simulink model "SCIM08"  (R2016a)
settings: Solver=FixedStepAuto  StartTime=0.0  StopTime=0.2  FixedStep=0.0001  RelTol=1e-3
values from neighbouring files (symbols this model uses):
  Lm = 0.1271    [motor4_workspace.mat]    (also in motor_wrapper.m = obj.Lm; scim_verifier.m = obj.motor.getLm(); setMotorParams.m; stationary_class.m = obj.Lm)
  Lr = 0.2744    [motor4_workspace.mat]    (also in motor_wrapper.m = obj.Lr; scim_verifier.m = obj.motor.getLr(); setMotorParams.m; stationary_class.m = obj.Lr)
  Ls = 0.2744    [motor4_workspace.mat]    (also in motor_wrapper.m = obj.Ls; scim_verifier.m = obj.motor.getLs(); setMotorParams.m; stationary.m = Ls/10)
  M_ab02abc = [1  0  1; -0.5  0.866025403784  1; -0.5  -0.866025403784  1]    [motor4_workspace.mat]    (also in setMotorParams.m = inv(M_abc2ab0); workspaceSav.mat)
  M_abc2ab0 = [0.666666666667  -0.333333333333  -0.333333333333; 0  0.57735026919  -0.57735026919; 0.333333333333  0.333333333333  0.333333333333]    [motor4_workspace.mat]    (also in setMotorParams.m = 2/3*[1, -0.5, -0.5; 0, sqrt(3)/2, -sqrt(3)/2;  0.5, 0.5, 0.5; workspaceSav.mat)
  Rr = 1.009    [motor4_workspace.mat]    (also in motor_wrapper.m = obj.Rr; setMotorParams.m; stationary_class.m = obj.Rr; stationary_from_eq.m = obj.Rr)
  sig = (tox-fromx)/6    [gaussSpace.m]    (also in motor4_workspace.mat = 0.785452782217; setMotorParams.m = 0.785452782217; stationary_class.m = 1-Lm*Lm/Ls/Lr; torqueFinder.m = 0.785452782217)
undefined symbols (not defined in the file or in its folder): Rows
libraries: simulink x1, dspsigops x1
settings Model: Creator=ebenera  LastModifiedBy=ebenera

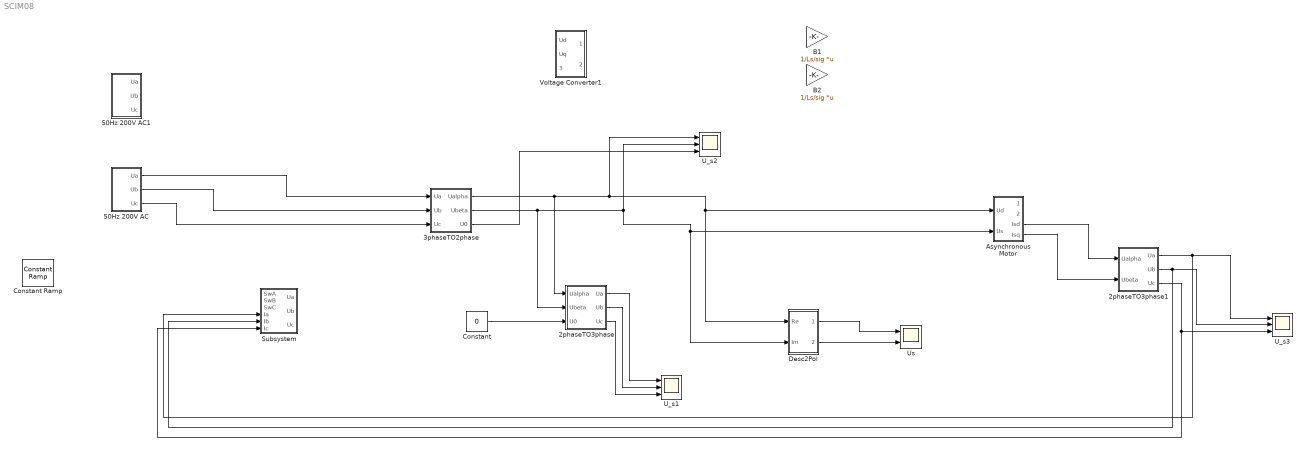
== system SCIM08 ==
  2phaseTO3phase : Subsystem
  2phaseTO3phase1 : Subsystem
  "3phaseTO2phase " : Subsystem
  50Hz 200V AC : Subsystem
  50Hz 200V AC1 : Subsystem
  Asynchronous Motor : Subsystem
  B1 : Gain  Gain=1/Ls/sig  Multiplication=Matrix(K*u)
  B2 : Gain  Gain=1/Ls/sig  Multiplication=Matrix(K*u)
  Constant : Constant  Value=0
  Constant Ramp : dspsigops/Constant Ramp  L=Rows  dim=1  Slope=1  dataType=Same as input  isSigned=on  wordLen=16  udDataType=sfix(16)  fracBitsMode=Best precision  numFracBits=15  Offset=0
  Desc2Pol : Subsystem
  Subsystem : Subsystem
  U_s1 : Scope  NumInputPorts=3
  U_s2 : Scope  NumInputPorts=3
  U_s3 : Scope  NumInputPorts=3
  Us : Scope  NumInputPorts=2
  Voltage Converter1 : Subsystem
  wires:
  "3phaseTO2phase "/1(Ualpha) -> 2phaseTO3phase/1(Ualpha), U_s2/1, Desc2Pol/1(Re), Asynchronous Motor/1(Ud)
  "3phaseTO2phase "/2(Ubeta) -> 2phaseTO3phase/2(Ubeta), Asynchronous Motor/2(Us), Desc2Pol/2(Im), U_s2/2
  Desc2Pol/1(Amp) -> Us/1
  Desc2Pol/2(Angle) -> Us/2
  "3phaseTO2phase "/3(U0) -> U_s2/3
  Constant/1 -> 2phaseTO3phase/3(U0)
  2phaseTO3phase/1(Ua) -> U_s1/1
  2phaseTO3phase/2(Ub) -> U_s1/2
  2phaseTO3phase/3(Uc) -> U_s1/3
  Asynchronous Motor/4(Isq) -> 2phaseTO3phase1/2(Ubeta)
  Asynchronous Motor/3(Isd) -> 2phaseTO3phase1/1(Ualpha)
  2phaseTO3phase1/1(Ua) -> Subsystem/4(Ia), U_s3/1
  2phaseTO3phase1/2(Ub) -> Subsystem/5(Ib), U_s3/2
  2phaseTO3phase1/3(Uc) -> Subsystem/6(Ic), U_s3/3
  50Hz 200V AC/1(Ua) -> "3phaseTO2phase "/1(Ua)
  50Hz 200V AC/2(Ub) -> "3phaseTO2phase "/2(Ub)
  50Hz 200V AC/3(Uc) -> "3phaseTO2phase "/3(Uc)

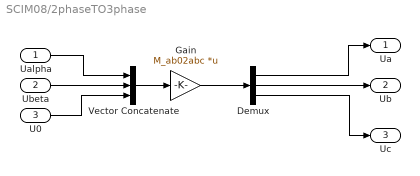
== system SCIM08/2phaseTO3phase ==
  Ualpha : Inport
  Ubeta : Inport  Port=2
  U0 : Inport  Port=3
  Demux : Demux  Outputs=3
  Gain : Gain  Gain=M_ab02abc  Multiplication=Matrix(K*u)
  Vector Concatenate : Concatenate  NumInputs=3
  Ua : Outport
  Ub : Outport  Port=2
  Uc : Outport  Port=3
  wires:
  Vector Concatenate/1 -> Gain/1
  Ualpha/1 -> Vector Concatenate/1
  Demux/3 -> Uc/1
  Gain/1 -> Demux/1
  U0/1 -> Vector Concatenate/3
  Ubeta/1 -> Vector Concatenate/2
  Demux/1 -> Ua/1
  Demux/2 -> Ub/1

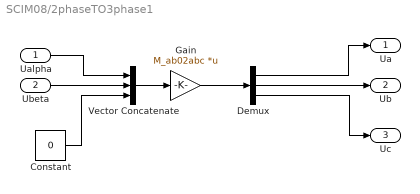
== system SCIM08/2phaseTO3phase1 ==
  Ualpha : Inport
  Ubeta : Inport  Port=2
  Constant : Constant  Value=0
  Demux : Demux  Outputs=3
  Gain : Gain  Gain=M_ab02abc  Multiplication=Matrix(K*u)
  Vector Concatenate : Concatenate  NumInputs=3
  Ua : Outport
  Ub : Outport  Port=2
  Uc : Outport  Port=3
  wires:
  Vector Concatenate/1 -> Gain/1
  Ualpha/1 -> Vector Concatenate/1
  Demux/3 -> Uc/1
  Gain/1 -> Demux/1
  Constant/1 -> Vector Concatenate/3
  Ubeta/1 -> Vector Concatenate/2
  Demux/1 -> Ua/1
  Demux/2 -> Ub/1

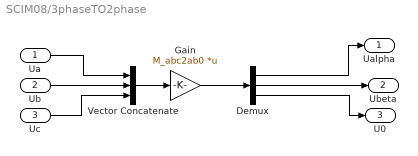
== system SCIM08/3phaseTO2phase  ==
  Ua : Inport
  Ub : Inport  Port=2
  Uc : Inport  Port=3
  Demux : Demux  Outputs=3
  Gain : Gain  Gain=M_abc2ab0  Multiplication=Matrix(K*u)
  Vector Concatenate : Concatenate  NumInputs=3
  Ualpha : Outport
  Ubeta : Outport  Port=2
  U0 : Outport  Port=3
  wires:
  Vector Concatenate/1 -> Gain/1
  Ua/1 -> Vector Concatenate/1
  Demux/3 -> U0/1
  Gain/1 -> Demux/1
  Uc/1 -> Vector Concatenate/3
  Ub/1 -> Vector Concatenate/2
  Demux/1 -> Ualpha/1
  Demux/2 -> Ubeta/1

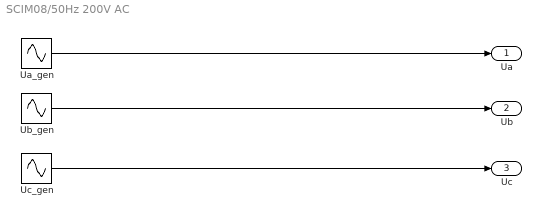
== system SCIM08/50Hz 200V AC ==
  Ua_gen : Sin  Amplitude=200  Frequency=314  SampleTime=0
  Ub_gen : Sin  Amplitude=200  Frequency=314  Phase=-2*pi/3  SampleTime=0
  Uc_gen : Sin  Amplitude=200  Frequency=314  Phase=2*pi/3  SampleTime=0
  Ua : Outport
  Ub : Outport  Port=2
  Uc : Outport  Port=3
  wires:
  Uc_gen/1 -> Uc/1
  Ub_gen/1 -> Ub/1
  Ua_gen/1 -> Ua/1

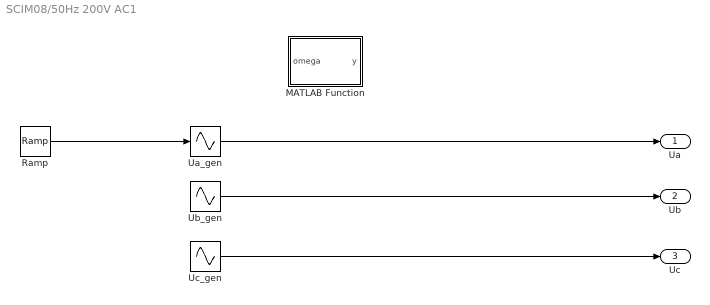
== system SCIM08/50Hz 200V AC1 ==
  MATLAB Function : MATLAB Function  TreatAsAtomicUnit=on
  Ramp : simulink/Sources/Ramp  slope=1  start=0  X0=0
  Ua_gen : Sin  TimeSource=Use external signal  Amplitude=200  Frequency=314  SampleTime=0
  Ub_gen : Sin  TimeSource=Use external signal  Amplitude=200  Frequency=314  Phase=-2*pi/3  SampleTime=0
  Uc_gen : Sin  TimeSource=Use external signal  Amplitude=200  Frequency=314  Phase=2*pi/3  SampleTime=0
  Ua : Outport
  Ub : Outport  Port=2
  Uc : Outport  Port=3
  wires:
  Uc_gen/1 -> Uc/1
  Ub_gen/1 -> Ub/1
  Ua_gen/1 -> Ua/1
  Ramp/1 -> Ua_gen/1
  ? -> Ub_gen/1

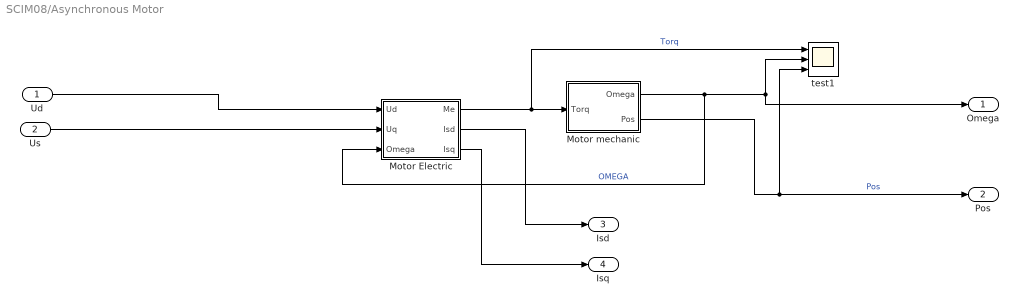
== system SCIM08/Asynchronous Motor ==
  Ud : Inport
  Us : Inport  Port=2
  Motor Electric : Subsystem
  Motor mechanic : Subsystem
  test1 : Scope  NumInputPorts=3
  Omega : Outport
  Pos : Outport  Port=2
  Isd : Outport  Port=3
  Isq : Outport  Port=4
  wires:
  Motor mechanic/2(Pos) -> test1/3, Pos/1  "Pos"
  Motor mechanic/1(Omega) -> test1/2, Omega/1, Motor Electric/3(Omega)  "OMEGA"
  Motor Electric/1(Me) -> test1/1, Motor mechanic/1("Torq ")  "Torq"
  Motor Electric/2(Isd) -> Isd/1
  Motor Electric/3(Isq) -> Isq/1
  Us/1 -> Motor Electric/2(Uq)
  Ud/1 -> Motor Electric/1(Ud)

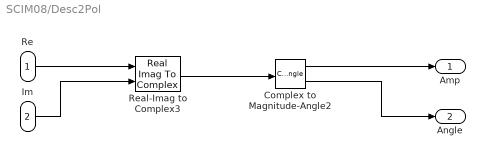
== system SCIM08/Desc2Pol ==
  Re : Inport
  Im : Inport  Port=2
  Complex to Magnitude-Angle2 : ComplexToMagnitudeAngle
  Real-Imag to Complex3 : RealImagToComplex
  Amp : Outport
  Angle : Outport  Port=2
  wires:
  Complex to Magnitude-Angle2/1 -> Amp/1
  Real-Imag to Complex3/1 -> Complex to Magnitude-Angle2/1
  Complex to Magnitude-Angle2/2 -> Angle/1
  Re/1 -> Real-Imag to Complex3/1
  Im/1 -> Real-Imag to Complex3/2

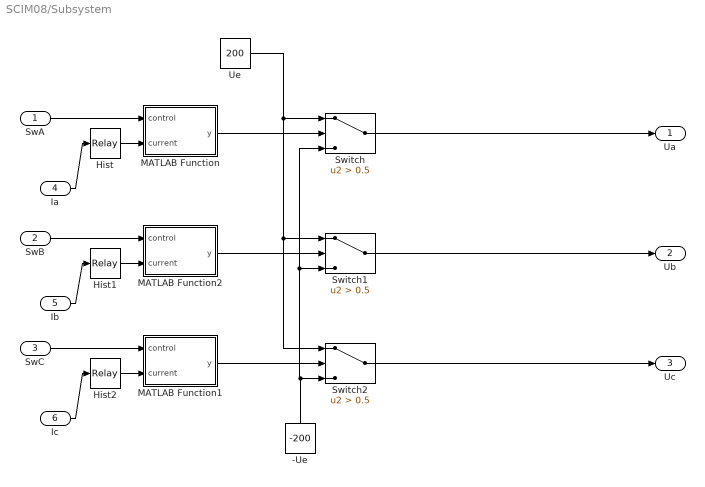
== system SCIM08/Subsystem ==
  SwA : Inport
  SwB : Inport  Port=2
  SwC : Inport  Port=3
  Ia : Inport  Port=4
  Ib : Inport  Port=5
  Ic : Inport  Port=6
  -Ue : Constant  Value=-200
  Hist : Relay  OnSwitchValue=0.1  OffSwitchValue=-0.5  OffOutputValue=-1
  Hist1 : Relay  OnSwitchValue=0.1  OffSwitchValue=-0.5  OffOutputValue=-1
  Hist2 : Relay  OnSwitchValue=0.1  OffSwitchValue=-0.5  OffOutputValue=-1
  MATLAB Function : MATLAB Function  TreatAsAtomicUnit=on
  MATLAB Function1 : MATLAB Function  TreatAsAtomicUnit=on
  MATLAB Function2 : MATLAB Function  TreatAsAtomicUnit=on
  Switch : Switch  Criteria=u2 > Threshold  Threshold=0.5
  Switch1 : Switch  Criteria=u2 > Threshold  Threshold=0.5
  Switch2 : Switch  Criteria=u2 > Threshold  Threshold=0.5
  Ue : Constant  Value=200
  Ua : Outport
  Ub : Outport  Port=2
  Uc : Outport  Port=3
  wires:
  -Ue/1 -> Switch/3, Switch1/3, Switch2/3
  Switch/1 -> Ua/1
  Ue/1 -> Switch2/1, Switch1/1, Switch/1
  Switch1/1 -> Ub/1
  Switch2/1 -> Uc/1
  MATLAB Function/1(y) -> Switch/2
  MATLAB Function2/1(y) -> Switch1/2
  MATLAB Function1/1(y) -> Switch2/2
  SwB/1 -> MATLAB Function2/1(control)
  SwA/1 -> MATLAB Function/1(control)
  SwC/1 -> MATLAB Function1/1(control)
  Ia/1 -> Hist/1
  Hist/1 -> MATLAB Function/2(current)
  Ib/1 -> Hist1/1
  Hist1/1 -> MATLAB Function2/2(current)
  Hist2/1 -> MATLAB Function1/2(current)
  Ic/1 -> Hist2/1

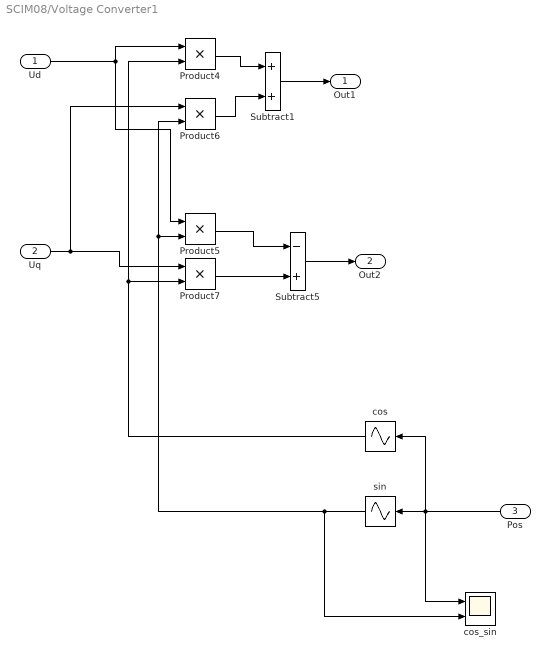
== system SCIM08/Voltage Converter1 ==
  Ud : Inport
  Uq : Inport  Port=2
  Pos : Inport  Port=3
  Product{4..7} (4 alike) : Product
  Subtract1 : Sum
  Subtract5 : Sum  Inputs=-+
  cos : Sin  TimeSource=Use external signal  Phase=+pi/2  SampleTime=0
  cos_sin : Scope  NumInputPorts=2
  sin : Sin  TimeSource=Use external signal  SampleTime=0
  Out1 : Outport
  Out2 : Outport  Port=2
  wires:
  cos/1 -> Product7/2, Product4/2
  Uq/1 -> Product6/1, Product7/1
  Ud/1 -> Product5/1, Product4/1
  Product4/1 -> Subtract1/1
  Product6/1 -> Subtract1/2
  Product5/1 -> Subtract5/1
  Product7/1 -> Subtract5/2
  Subtract5/1 -> Out2/1
  Subtract1/1 -> Out1/1
  sin/1 -> Product5/2, Product6/2, cos_sin/2
  Pos/1 -> cos_sin/1, sin/1, cos/1

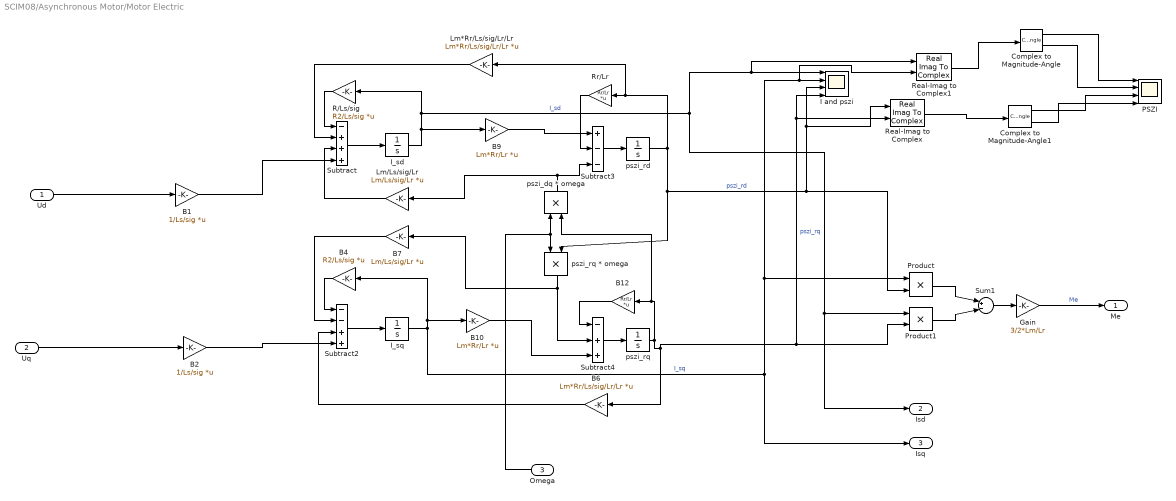
== system SCIM08/Asynchronous Motor/Motor Electric ==
  Ud : Inport
  Uq : Inport  Port=2
  Omega : Inport  Port=3
  B1 : Gain  Gain=1/Ls/sig  Multiplication=Matrix(K*u)
  B10 : Gain  Gain=Lm*Rr/Lr  Multiplication=Matrix(K*u)
  B12 : Gain  Gain=Rr/Lr  Multiplication=Matrix(K*u)
  B2 : Gain  Gain=1/Ls/sig  Multiplication=Matrix(K*u)
  B4 : Gain  Gain=R2/Ls/sig  Multiplication=Matrix(K*u)
  B6 : Gain  Gain=Lm*Rr/Ls/sig/Lr/Lr  Multiplication=Matrix(K*u)
  B7 : Gain  Gain=Lm/Ls/sig/Lr  Multiplication=Matrix(K*u)
  B9 : Gain  Gain=Lm*Rr/Lr  Multiplication=Matrix(K*u)
  Complex to Magnitude-Angle : ComplexToMagnitudeAngle
  Complex to Magnitude-Angle1 : ComplexToMagnitudeAngle
  Gain : Gain  Gain=3/2*Lm/Lr
  I and pszi : Scope  NumInputPorts=4
  I_sd : Integrator
  I_sq : Integrator
  Lm*Rr/Ls/sig/Lr/Lr : Gain  Gain=Lm*Rr/Ls/sig/Lr/Lr  Multiplication=Matrix(K*u)
  Lm/Ls/sig/Lr : Gain  Gain=Lm/Ls/sig/Lr  Multiplication=Matrix(K*u)
  PSZI : Scope  NumInputPorts=4
  Product : Product
  Product1 : Product
  R/Ls/sig : Gain  Gain=R2/Ls/sig  Multiplication=Matrix(K*u)
  Real-Imag to Complex : RealImagToComplex
  Real-Imag to Complex1 : RealImagToComplex
  Rr/Lr : Gain  Gain=Rr/Lr  Multiplication=Matrix(K*u)
  Subtract : Sum  Inputs=-+++
  Subtract2 : Sum  Inputs=--++
  Subtract3 : Sum  Inputs=+--
  Subtract4 : Sum  Inputs=-++
  Sum1 : Sum  Inputs=|+-|
  pszi_dq * omega : Product
  pszi_rd : Integrator
  "pszi_rq " : Integrator
  pszi_rq * omega : Product
  Me : Outport
  Isd : Outport  Port=2
  Isq : Outport  Port=3
  wires:
  pszi_rq * omega/1 -> Subtract4/2, B7/1
  Subtract/1 -> I_sd/1
  B12/1 -> Subtract4/1
  Product1/1 -> Sum1/2
  Lm*Rr/Ls/sig/Lr/Lr/1 -> Subtract/2
  Product/1 -> Sum1/1
  I_sq/1 -> Isq/1, Real-Imag to Complex1/2, I and pszi/2, Product/1, B10/1, B4/1  "I_sq"
  I_sd/1 -> B9/1, Isd/1, Product1/1, Real-Imag to Complex1/1, I and pszi/1, R/Ls/sig/1  "I_sd"
  Sum1/1 -> Gain/1
  R/Ls/sig/1 -> Subtract/1
  B6/1 -> Subtract2/3
  B4/1 -> Subtract2/1
  pszi_dq * omega/1 -> Subtract3/3, Lm/Ls/sig/Lr/1
  Omega/1 -> pszi_rq * omega/1, pszi_dq * omega/1
  B9/1 -> Subtract3/1
  Rr/Lr/1 -> Subtract3/2
  pszi_rd/1 -> Real-Imag to Complex/1, I and pszi/3, Product/2, pszi_rq * omega/2, Lm*Rr/Ls/sig/Lr/Lr/1, Rr/Lr/1  "pszi_rd"
  Lm/Ls/sig/Lr/1 -> Subtract/3
  "pszi_rq "/1 -> pszi_dq * omega/2, B12/1, Real-Imag to Complex/2, I and pszi/4, Product1/2, B6/1  "pszi_rq"
  B7/1 -> Subtract2/2
  Gain/1 -> Me/1  "Me"
  B10/1 -> Subtract4/3
  Subtract4/1 -> "pszi_rq "/1
  Subtract2/1 -> I_sq/1
  Subtract3/1 -> pszi_rd/1
  Uq/1 -> B2/1
  Ud/1 -> B1/1
  B1/1 -> Subtract/4
  B2/1 -> Subtract2/4
  Real-Imag to Complex1/1 -> Complex to Magnitude-Angle/1
  Complex to Magnitude-Angle/1 -> PSZI/1
  Complex to Magnitude-Angle/2 -> PSZI/2
  Real-Imag to Complex/1 -> Complex to Magnitude-Angle1/1
  Complex to Magnitude-Angle1/1 -> PSZI/3
  Complex to Magnitude-Angle1/2 -> PSZI/4

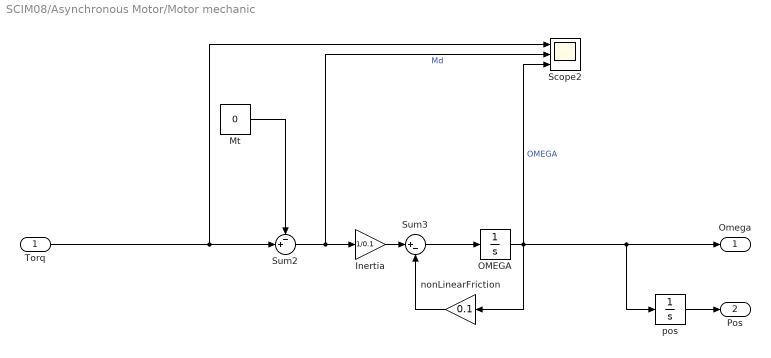
== system SCIM08/Asynchronous Motor/Motor mechanic ==
  "Torq " : Inport
  Inertia : Gain  Gain=1/0.1
  Mt : Constant  Value=0
  OMEGA : Integrator
  Scope2 : Scope  NumInputPorts=3
  Sum2 : Sum  Inputs=-+|
  Sum3 : Sum  Inputs=|+-
  nonLinearFriction : Gain  Gain=0.1
  pos : Integrator  WrapState=on
  Omega : Outport
  Pos : Outport  Port=2
  wires:
  "Torq "/1 -> Scope2/1, Sum2/2
  OMEGA/1 -> Scope2/3, pos/1, Omega/1, nonLinearFriction/1  "OMEGA"
  Sum3/1 -> OMEGA/1
  Sum2/1 -> Inertia/1, Scope2/2  "Md"
  Mt/1 -> Sum2/1
  nonLinearFriction/1 -> Sum3/2
  Inertia/1 -> Sum3/1
  pos/1 -> Pos/1

== matlab function SCIM08/Subsystem/MATLAB Function1 ==
  data: control input; y output; current input
function y = fcn(control, current)
	if control >= 1
        y = 1;
    elseif control <= -1
        y=-1;
    elseif(current>0)
        y = -1;
    else
        y = 1;
    end
end

== matlab function SCIM08/Subsystem/MATLAB Function ==
  data: control input; y output; current input
function y = fcn(control, current)
	if control >= 1
        y = 1;
    elseif control <= -1
        y=-1;
    elseif(current>0)
        y = -1;
    else
        y = 1;
    end
end

== matlab function SCIM08/Subsystem/MATLAB Function2 ==
  data: control input; y output; current input
function y = fcn(control, current)
	if control >= 1
        y = 1;
    elseif control <= -1
        y=-1;
    elseif(current>0)
        y = -1;
    else
        y = 1;
    end
end

== matlab function SCIM08/50Hz 200V AC1/MATLAB Function ==
  data: omega input; y output
function y = fcn(omega)
%#codegen
    persistent phase = 0;
    SampleTime = get_param(MdlName,'FixedStep');
    

y = u;
